simulink model "Periptwsi_1"  (R2020a)
settings: Solver=VariableStepAuto  StartTime=0.0  StopTime=20  RelTol=1e-3
libraries: fuzblock x2, simulink x1
settings Model: Creator=Vasilis Kyrgyrides  LastModifiedBy=Vasilis Kyrgyrides

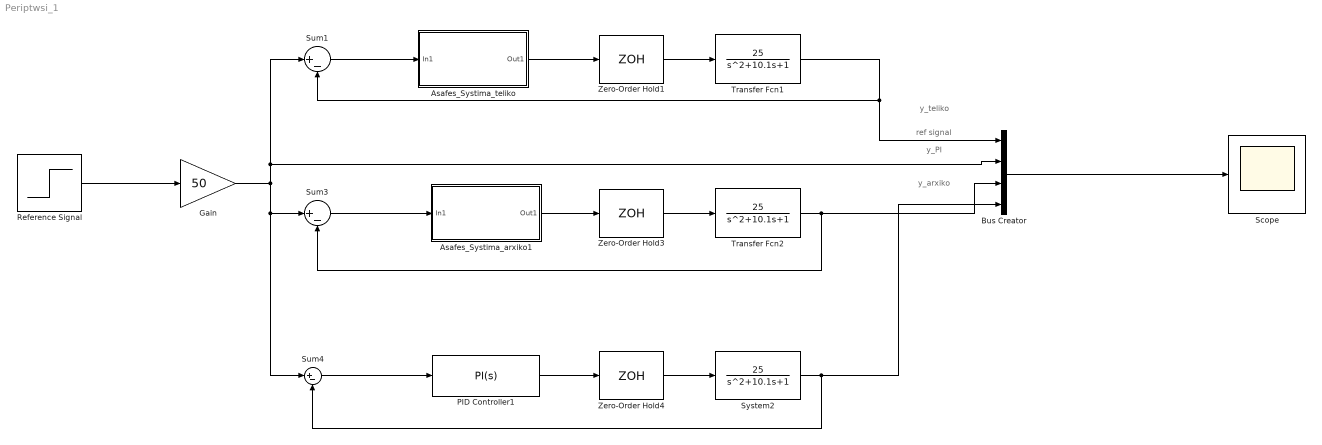
== system Periptwsi_1 ==
  note: y_PI
  note: ref signal
  note: y_teliko
  note: y_arxiko
  Asafes_Systima_arxiko1 : Subsystem
  Asafes_Systima_teliko : Subsystem
  Bus Creator : BusCreator  Inputs=4
  Gain : Gain  Gain=50
  PID Controller1 : simulink/Continuous/PID Controller  Controller=PI  Form=Parallel  TimeDomain=Continuous-time  UseExternalTs=off  SampleTime=-1  IntegratorMethod=Forward Euler  FilterMethod=Forward Euler  ControllerParametersSource=internal  P=1.262  I=0.36598  D=0.02  UseFilter=on  N=20  TunerSelectOption=Transfer Function Based (PID Tuner App)  InitialConditionSource=internal  InitialConditionForIntegrator=0  InitialConditionForFilter=0  DifferentiatorICPrevScaledInput=0  ExternalReset=none  TrackingMode=off  Kt=1  LimitOutput=off  UpperSaturationLimit=inf  LowerSaturationLimit=-inf  LinearizeAsGain=on  AntiWindupMode=none  Kb=1  POutMin=[]  POutMax=[]  IOutMin=[]  IOutMax=[]  DOutMin=[]  DOutMax=[]  NOutMin=[]  NOutMax=[]  SumOutMin=[]  SumOutMax=[]  SaturationOutMin=[]  SaturationOutMax=[]  PParamMin=[]  PParamMax=[]  IParamMin=[]  IParamMax=[]  DParamMin=[]  DParamMax=[]  NParamMin=[]  NParamMax=[]  KbParamMin=[]  KbParamMax=[]  KtParamMin=[]  KtParamMax=[]  KbOutMin=[]  KbOutMax=[]  KtOutMin=[]  KtOutMax=[]  IntegratorOutMin=[]  IntegratorOutMax=[]  FilterOutMin=[]  FilterOutMax=[]  SumI1OutMin=[]  SumI1OutMax=[]  SumI2OutMin=[]  SumI2OutMax=[]  SumI3OutMin=[]  SumI3OutMax=[]  SumI4OutMin=[]  SumI4OutMax=[]  SumDOutMin=[]  SumDOutMax=[]  DifferentiatorOutMin=[]  DifferentiatorOutMax=[]  FilterDiffOutCoefMin=[]  FilterDiffOutCoefMax=[]  ReciprocalOutMin=[]  ReciprocalOutMax=[]  SumDenOutMin=[]  SumDenOutMax=[]  SumNumOutMin=[]  SumNumOutMax=[]  DivideOutMin=[]  DivideOutMax=[]  UdiffTsProdOutMin=[]  UdiffTsProdOutMax=[]  NTsProdOutMin=[]  NTsProdOutMax=[]  UintegralTsProdOutMin=[]  UintegralTsProdOutMax=[]  UngainTsProdOutMin=[]  UngainTsProdOutMax=[]  IntegratorContinuousStateAttributes=''  IntegratorStateMustResolveToSignalObject=off  IntegratorRTWStateStorageClass=Auto  FilterContinuousStateAttributes=''  FilterStateMustResolveToSignalObject=off  FilterRTWStateStorageClass=Auto  ParallelPVariant=InternalParameters  IdealPVariant=Disabled  IVariant=InternalParameters  DVariant=Disabled  IntegratorVariant=Continuous  SatVariant=Disabled  AWVariant=Passthrough  PCopyVariant=Disabled  TRVariant=Disabled  FdbkBlocksVariant=Forward  IdealPFdbkVariant=Disabled  SatFdbkVariant=Disabled  DerivativeFilterVariant=Disabled  NVariant=Disabled  NCopyVariant=Disabled_SignalSpec  FilterICVariant=Disabled  IntegratorICVariant=InternalICs  ExternalResetVariant=Disabled  TRSumVariant=Passthrough  SumFdbkVariant=Disabled  SumVariant=Sum_PI  TsampFilterVariant=InternalTs  TsampNgainVariant=Passthrough  TsampIntegralVariant=Passthrough
  Reference Signal : Step  Time=0  SampleTime=0.01
  Scope : Scope
  Sum1 : Sum  Inputs=|+-
  Sum3 : Sum  Inputs=|+-
  Sum4 : Sum  Inputs=|+-
  System2 : TransferFcn  Numerator=[25]  Denominator=[1 10.1 1]
  Transfer Fcn1 : TransferFcn  Numerator=[25]  Denominator=[1 10.1 1]
  Transfer Fcn2 : TransferFcn  Numerator=[25]  Denominator=[1 10.1 1]
  Zero-Order Hold1 : ZeroOrderHold  SampleTime=-1
  Zero-Order Hold3 : ZeroOrderHold  SampleTime=-1
  Zero-Order Hold4 : ZeroOrderHold  SampleTime=-1
  wires:
  Reference Signal/1 -> Gain/1
  Asafes_Systima_teliko/1(Out1) -> Zero-Order Hold1/1
  Zero-Order Hold1/1 -> Transfer Fcn1/1
  Transfer Fcn1/1 -> Bus Creator/1, Sum1/2
  Sum1/1 -> Asafes_Systima_teliko/1(In1)
  Zero-Order Hold4/1 -> System2/1
  PID Controller1/1 -> Zero-Order Hold4/1
  Sum3/1 -> Asafes_Systima_arxiko1/1(In1)
  Sum4/1 -> PID Controller1/1
  Transfer Fcn2/1 -> Bus Creator/3, Sum3/2
  Asafes_Systima_arxiko1/1(Out1) -> Zero-Order Hold3/1
  Zero-Order Hold3/1 -> Transfer Fcn2/1
  System2/1 -> Bus Creator/4, Sum4/2
  Bus Creator/1 -> Scope/1
  Gain/1 -> Sum1/1, Bus Creator/2, Sum4/1, Sum3/1

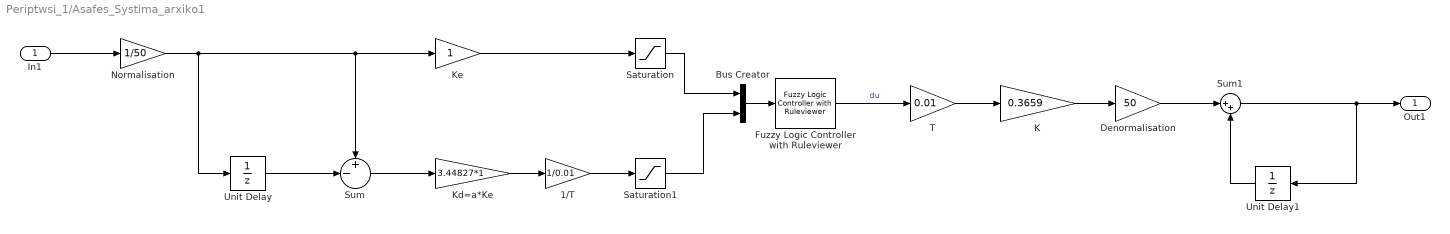
== system Periptwsi_1/Asafes_Systima_arxiko1 ==
  In1 : Inport
  1/T : Gain  Gain=1/0.01
  Bus Creator : BusCreator  Inputs=2
  Denormalisation : Gain  Gain=50
  Fuzzy Logic Controller with Ruleviewer : fuzblock/Fuzzy Logic  Controller  with Ruleviewer  fismatrix=Asafis_PI_2  Ts=0.01
  K : Gain  Gain=0.3659
  Kd=a*Ke : Gain  Gain=3.44827*1
  Ke : Gain
  Normalisation : Gain  Gain=1/50
  Saturation : Saturate  UpperLimit=1  LowerLimit=-1
  Saturation1 : Saturate  UpperLimit=1  LowerLimit=-1
  Sum : Sum  Inputs=+-|
  Sum1 : Sum  Inputs=|++
  T : Gain  Gain=0.01
  Unit Delay : UnitDelay  SampleTime=-1  HasFrameUpgradeWarning=on
  Unit Delay1 : UnitDelay  SampleTime=-1  HasFrameUpgradeWarning=on
  Out1 : Outport
  wires:
  In1/1 -> Normalisation/1
  Unit Delay/1 -> Sum/2
  Normalisation/1 -> Sum/1, Ke/1, Unit Delay/1
  Sum/1 -> Kd=a*Ke/1
  Kd=a*Ke/1 -> 1/T/1
  Ke/1 -> Saturation/1
  1/T/1 -> Saturation1/1
  Saturation1/1 -> Bus Creator/2
  Saturation/1 -> Bus Creator/1
  K/1 -> Denormalisation/1
  T/1 -> K/1
  Fuzzy Logic Controller with Ruleviewer/1 -> T/1  "du"
  Denormalisation/1 -> Sum1/1
  Sum1/1 -> Unit Delay1/1, Out1/1
  Unit Delay1/1 -> Sum1/2
  Bus Creator/1 -> Fuzzy Logic Controller with Ruleviewer/1

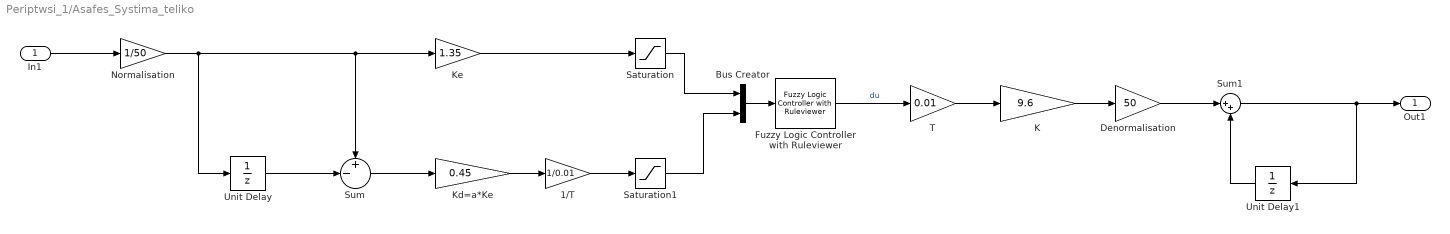
== system Periptwsi_1/Asafes_Systima_teliko ==
  In1 : Inport
  1/T : Gain  Gain=1/0.01
  Bus Creator : BusCreator  Inputs=2
  Denormalisation : Gain  Gain=50
  Fuzzy Logic Controller with Ruleviewer : fuzblock/Fuzzy Logic  Controller  with Ruleviewer  fismatrix=Asafis_PI_2  Ts=0.01
  K : Gain  Gain=9.6
  Kd=a*Ke : Gain  Gain=0.45
  Ke : Gain  Gain=1.35
  Normalisation : Gain  Gain=1/50
  Saturation : Saturate  UpperLimit=1  LowerLimit=-1
  Saturation1 : Saturate  UpperLimit=1  LowerLimit=-1
  Sum : Sum  Inputs=+-|
  Sum1 : Sum  Inputs=|++
  T : Gain  Gain=0.01
  Unit Delay : UnitDelay  SampleTime=-1  HasFrameUpgradeWarning=on
  Unit Delay1 : UnitDelay  SampleTime=-1  HasFrameUpgradeWarning=on
  Out1 : Outport
  wires:
  In1/1 -> Normalisation/1
  Unit Delay/1 -> Sum/2
  Normalisation/1 -> Sum/1, Ke/1, Unit Delay/1
  Sum/1 -> Kd=a*Ke/1
  Kd=a*Ke/1 -> 1/T/1
  Ke/1 -> Saturation/1
  1/T/1 -> Saturation1/1
  Saturation1/1 -> Bus Creator/2
  Saturation/1 -> Bus Creator/1
  K/1 -> Denormalisation/1
  T/1 -> K/1
  Fuzzy Logic Controller with Ruleviewer/1 -> T/1  "du"
  Denormalisation/1 -> Sum1/1
  Sum1/1 -> Unit Delay1/1, Out1/1
  Unit Delay1/1 -> Sum1/2
  Bus Creator/1 -> Fuzzy Logic Controller with Ruleviewer/1
